simulink model "UrbanCHIL"  (Simulink 8.1)
settings: Solver=ode1  StartTime=0.0  StopTime=inf  FixedStep=Ts  MaxStep=1e-3  RelTol=1e-3
PostLoadFcn:
  | NREL_Mode=1; BANSHEE_init;
InitFcn:
  | NREL_Mode=1; BANSHEE_init;
values from neighbouring files (symbols this model uses):
  DER_REL = xlsread('DER_relay.xlsx')    [relay_settings_init.m]
  F0 = xlsread('F0_relay_banshee.xlsx')    [relay_settings_init.m]
  F2 = xlsread('F2_relay_banshee.xlsx')    [relay_settings_init.m]
  F3 = xlsread('F3_relay_banshee.xlsx')    [relay_settings_init.m]
  F4 = xlsread('F4_relay_nrel.xlsx')    [relay_settings_init.m]
  Ts = 100E-6    (= 0.0001)    [BANSHEE_init.m]    (also in Ghost_init.m)
undefined symbols (not defined in the file or in its folder): CBID, communications_lib, Feeder2_lib, Feeder3_lib, Feeder4_lib, generic_ethernet_cb, Left, relay_housing_lib, SM_UtilityService, SS_COMMUNICATION, SS_F2_RELAY_HOUSING, SS_F3_RELAY_HOUSING, SS_Feeder2, SS_Feeder3, SS_Feeder4, Stim, type, utility_service_lib, V
libraries: simulink x80, relay_modbus_lib x80, breaker_lib x46, rtio_generic_modbus x45, cables_lib x30, rtlab x22, Load_lib x21, powerlib x20, transformer_lib x19, ssn_lib x13, artemis x6, BESS_lib x4
(part 2 of 6)

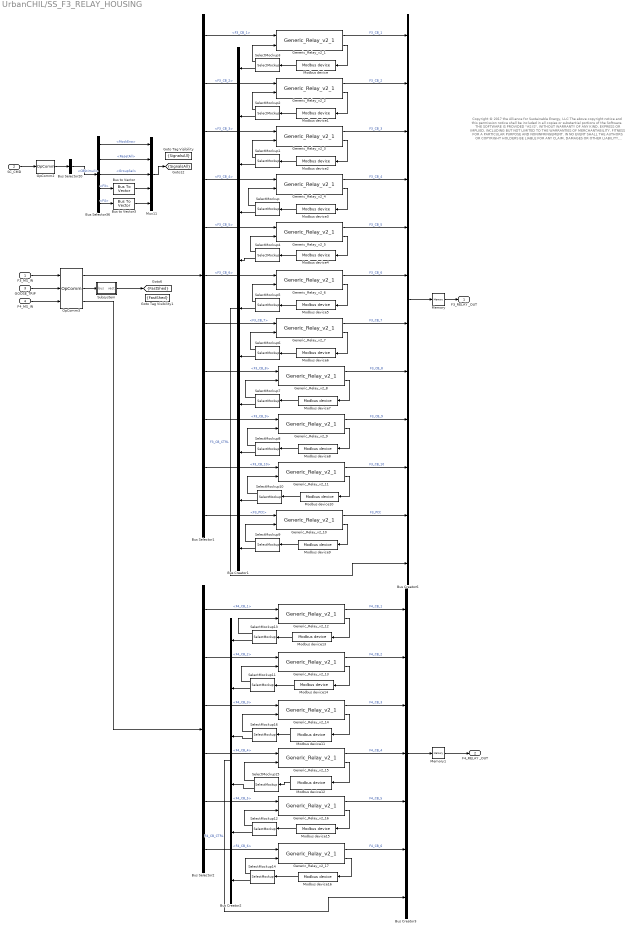
== system UrbanCHIL/SS_F3_RELAY_HOUSING ==
  note: Copyright © 2017 the Alliance for Sustainable Energy, LLC
      |
      | The above copyright notice and this permission notice shall be included in all copies or substantial portions of the Software.
      |
      | THE SOFTWARE IS PROVIDED "AS IS", WITHOUT WARRANTY OF ANY KIND, EXPRESS OR IMPLIED, INCLUDING
      | BUT NOT LIMITED TO THE WARRANTIES OF MERCHANTABILITY, FITNESS FOR A PARTICULAR PURPOSE AND
      | NONINFRINGEMENT. IN NO EVENT SHALL THE AUTHORS OR COPYRIGHT HOLDERS BE LIABLE FOR ANY CLAIM,
      |  DAMAGES OR OTHER LIABILITY, WHETHER IN AN ACTION OF CONTRACT, TORT OR OTHERWISE, ARISING FROM,
      | OUT OF OR IN CONNECTION WITH THE SOFTWARE OR THE USE OR OTHER DEALINGS IN THE SOFTWARE
  F3_MS_IN : Inport
  SC_CMD : Inport  Port=2
  GOOSE_TRIP : Inport  Port=3
  F4_MS_IN : Inport  Port=4
  Bus Creator1 : BusCreator  Inputs=11
  Bus Creator2 : BusCreator  Inputs=6
  Bus Creator3 : BusCreator  Inputs=7
  Bus Creator6 : BusCreator  Inputs=12
  Bus Selector1 : BusSelector  OutputSignals=CB_DATA.F3_CB_1,CB_DATA.F3_CB_2,CB_DATA.F3_CB_3,CB_DATA.F3_CB_4,CB_DATA.F3_CB_5,CB_DATA.F3_CB_6,CB_DATA.F3_CB_7,CB_DATA.F3_CB_8,CB_DATA.F3_CB_9,CB_DATA.F3_CB_10,CB_DATA.F3_PCC
  Bus Selector2 : BusSelector  OutputSignals=CB_DATA.F4_CB_1,CB_DATA.F4_CB_2,CB_DATA.F4_CB_3,CB_DATA.F4_CB_4,CB_DATA.F4_CB_5,CB_DATA.F4_CB_6
  Bus Selector20 : BusSelector  OutputSignals=CBStimuli
  Bus Selector36 : BusSelector  OutputSignals=MockEna,ResetAll,GroupSel,F3,F4
  Bus to Vector : BusToVector
  Bus to Vector3 : BusToVector
  Generic_Relay_v2_1 : relay_modbus_lib/Generic_Relay_v2_1  Ts=Ts  relay_settings=[F3(1,:)]
  Generic_Relay_v2_10 : relay_modbus_lib/Generic_Relay_v2_1  Ts=Ts  relay_settings=[F0(3,:)]
  Generic_Relay_v2_11 : relay_modbus_lib/Generic_Relay_v2_1  Ts=Ts  relay_settings=[F3(10,:)]
  Generic_Relay_v2_12 : relay_modbus_lib/Generic_Relay_v2_1  Ts=Ts  relay_settings=[F4(1,:)]
  Generic_Relay_v2_13 : relay_modbus_lib/Generic_Relay_v2_1  Ts=Ts  relay_settings=[F4(2,:)]
  Generic_Relay_v2_14 : relay_modbus_lib/Generic_Relay_v2_1  Ts=Ts  relay_settings=[F4(3,:)]
  Generic_Relay_v2_15 : relay_modbus_lib/Generic_Relay_v2_1  Ts=Ts  relay_settings=[F4(4,:)]
  Generic_Relay_v2_16 : relay_modbus_lib/Generic_Relay_v2_1  Ts=Ts  relay_settings=[F4(5,:)]
  Generic_Relay_v2_17 : relay_modbus_lib/Generic_Relay_v2_1  Ts=Ts  relay_settings=[F4(6,:)]
  Generic_Relay_v2_2 : relay_modbus_lib/Generic_Relay_v2_1  Ts=Ts  relay_settings=[F3(2,:)]
  Generic_Relay_v2_3 : relay_modbus_lib/Generic_Relay_v2_1  Ts=Ts  relay_settings=[F3(3,:)]
  Generic_Relay_v2_4 : relay_modbus_lib/Generic_Relay_v2_1  Ts=Ts  relay_settings=[F3(4,:)]
  Generic_Relay_v2_5 : relay_modbus_lib/Generic_Relay_v2_1  Ts=Ts  relay_settings=[F3(5,:)]
  Generic_Relay_v2_6 : relay_modbus_lib/Generic_Relay_v2_1  Ts=Ts  relay_settings=[F3(6,:)]
  Generic_Relay_v2_7 : relay_modbus_lib/Generic_Relay_v2_1  Ts=Ts  relay_settings=[F3(7,:)]
  Generic_Relay_v2_8 : relay_modbus_lib/Generic_Relay_v2_1  Ts=Ts  relay_settings=[F3(8,:)]
  Generic_Relay_v2_9 : relay_modbus_lib/Generic_Relay_v2_1  Ts=Ts  relay_settings=[F3(9,:)]
  Goto Tag Visibility : GotoTagVisibility  GotoTag=SignalsAll
  Goto Tag Visibility1 : GotoTagVisibility  GotoTag=FastShed
  Memory : Memory
  Memory1 : Memory
  Modbus device : rtio_generic_modbus/Modbus device  conf_name=F3_relay_cfg1.opal  conf_name_mask=F3_relay_cfg1.xls  sample_time=Ts
  Modbus device1 : rtio_generic_modbus/Modbus device  conf_name=F3_relay_cfg2.opal  conf_name_mask=F3_relay_cfg2.xls  sample_time=Ts
  Modbus device10 : rtio_generic_modbus/Modbus device  conf_name=F3_relay_cfg10.opal  conf_name_mask=F3_relay_cfg10.xls  sample_time=Ts
  Modbus device11 : rtio_generic_modbus/Modbus device  conf_name=F4_relay_cfg3.opal  conf_name_mask=F4_relay_cfg3.xls  sample_time=Ts
  Modbus device12 : rtio_generic_modbus/Modbus device  conf_name=F4_relay_cfg4.opal  conf_name_mask=F4_relay_cfg4.xls  sample_time=Ts
  Modbus device13 : rtio_generic_modbus/Modbus device  conf_name=F4_relay_cfg1.opal  conf_name_mask=F4_relay_cfg1.xls  sample_time=Ts
  Modbus device14 : rtio_generic_modbus/Modbus device  conf_name=F4_relay_cfg2.opal  conf_name_mask=F4_relay_cfg2.xls  sample_time=Ts
  Modbus device15 : rtio_generic_modbus/Modbus device  conf_name=F4_relay_cfg5.opal  conf_name_mask=F4_relay_cfg5.xls  sample_time=Ts
  Modbus device16 : rtio_generic_modbus/Modbus device  conf_name=F4_relay_cfg6.opal  conf_name_mask=F4_relay_cfg6.xls  sample_time=Ts
  Modbus device2 : rtio_generic_modbus/Modbus device  conf_name=F3_relay_cfg3.opal  conf_name_mask=F3_relay_cfg3.xls  sample_time=Ts
  Modbus device3 : rtio_generic_modbus/Modbus device  conf_name=F3_relay_cfg4.opal  conf_name_mask=F3_relay_cfg4.xls  sample_time=Ts
  Modbus device4 : rtio_generic_modbus/Modbus device  conf_name=F3_relay_cfg5.opal  conf_name_mask=F3_relay_cfg5.xls  sample_time=Ts
  Modbus device5 : rtio_generic_modbus/Modbus device  conf_name=F3_relay_cfg6.opal  conf_name_mask=F3_relay_cfg6.xls  sample_time=Ts
  Modbus device6 : rtio_generic_modbus/Modbus device  conf_name=F3_relay_cfg7.opal  conf_name_mask=F3_relay_cfg7.xls  sample_time=Ts
  Modbus device7 : rtio_generic_modbus/Modbus device  conf_name=F3_relay_cfg8.opal  conf_name_mask=F3_relay_cfg8.xls  sample_time=Ts
  Modbus device8 : rtio_generic_modbus/Modbus device  conf_name=F3_relay_cfg9.opal  conf_name_mask=F3_relay_cfg9.xls  sample_time=Ts
  Modbus device9 : rtio_generic_modbus/Modbus device  conf_name=F3_relay_cfg_pcc.opal  conf_name_mask=F3_relay_cfg_pcc.xls  sample_time=Ts
  Mux11 : Mux  Inputs=5
  OpComm2 : rtlab/OpComm  nbport=1  groupe_acq=1  subsys_rate=0  st=0  Synchronization=on  Interpolation=on  Threshold=1.0  Missed_Data=off  Sim_Time=off  Samples=off  dynSigOut=off  from_console=0  warning_done=off  writeOpCommFile=off  Offset=off
  OpComm3 : rtlab/OpComm  nbport=3  groupe_acq=1  subsys_rate=0  st=0  Synchronization=on  Interpolation=on  Threshold=1.0  Missed_Data=off  Sim_Time=off  Samples=off  dynSigOut=off  from_console=0  warning_done=off  writeOpCommFile=off  Offset=off
  SelectMockup : relay_modbus_lib/SelectMockup  sigID=4  sigN=17
  SelectMockup1 : relay_modbus_lib/SelectMockup  sigID=3  sigN=17
  SelectMockup10 : relay_modbus_lib/SelectMockup  sigID=10  sigN=17
  SelectMockup11 : relay_modbus_lib/SelectMockup  sigID=13  sigN=17
  SelectMockup12 : relay_modbus_lib/SelectMockup  sigID=16  sigN=17
  SelectMockup13 : relay_modbus_lib/SelectMockup  sigID=12  sigN=17
  SelectMockup14 : relay_modbus_lib/SelectMockup  sigID=17  sigN=17
  SelectMockup15 : relay_modbus_lib/SelectMockup  sigID=15  sigN=17
  SelectMockup16 : relay_modbus_lib/SelectMockup  sigID=14  sigN=17
  SelectMockup2 : relay_modbus_lib/SelectMockup  sigID=2  sigN=17
  SelectMockup3 : relay_modbus_lib/SelectMockup  sigID=1  sigN=17
  SelectMockup4 : relay_modbus_lib/SelectMockup  sigID=5  sigN=17
  SelectMockup5 : relay_modbus_lib/SelectMockup  sigID=6  sigN=17
  SelectMockup6 : relay_modbus_lib/SelectMockup  sigID=7  sigN=17
  SelectMockup7 : relay_modbus_lib/SelectMockup  sigID=8  sigN=17
  SelectMockup8 : relay_modbus_lib/SelectMockup  sigID=9  sigN=17
  SelectMockup9 : relay_modbus_lib/SelectMockup  sigID=11  sigN=17
  Subsystem : Subsystem
  F3_RELAY _OUT : Outport
  F4_RELAY _OUT : Outport  Port=2
  tag scope: FastShed=scoped, SignalsAll=scoped
  wires:
  OpComm3/1 -> Bus Selector1/1
  Generic_Relay_v2_1/2 -> Modbus device/1
  SelectMockup3/1 -> Generic_Relay_v2_1/2
  Generic_Relay_v2_2/2 -> Modbus device1/1
  SelectMockup2/1 -> Generic_Relay_v2_2/2
  SelectMockup1/1 -> Generic_Relay_v2_3/2
  Generic_Relay_v2_3/2 -> Modbus device2/1
  Generic_Relay_v2_4/2 -> Modbus device3/1
  SelectMockup/1 -> Generic_Relay_v2_4/2
  Generic_Relay_v2_5/2 -> Modbus device4/1
  SelectMockup4/1 -> Generic_Relay_v2_5/2
  SelectMockup5/1 -> Generic_Relay_v2_6/2
  Generic_Relay_v2_6/2 -> Modbus device5/1
  Generic_Relay_v2_7/2 -> Modbus device6/1
  SelectMockup6/1 -> Generic_Relay_v2_7/2
  F3_MS_IN/1 -> OpComm3/1
  Bus Selector1/1 -> Generic_Relay_v2_1/1  "<F3_CB_1>"
  Bus Selector1/2 -> Generic_Relay_v2_2/1  "<F3_CB_2>"
  Bus Selector1/3 -> Generic_Relay_v2_3/1  "<F3_CB_3>"
  Bus Selector1/4 -> Generic_Relay_v2_4/1  "<F3_CB_4>"
  Bus Selector1/5 -> Generic_Relay_v2_5/1  "<F3_CB_5>"
  Bus Selector1/6 -> Generic_Relay_v2_6/1  "<F3_CB_6>"
  Bus Selector1/7 -> Generic_Relay_v2_7/1  "<F3_CB_7>"
  Generic_Relay_v2_1/1 -> Bus Creator6/1  "F3_CB_1"
  Generic_Relay_v2_2/1 -> Bus Creator6/2  "F3_CB_2"
  Generic_Relay_v2_3/1 -> Bus Creator6/3  "F3_CB_3"
  Generic_Relay_v2_4/1 -> Bus Creator6/4  "F3_CB_4"
  Generic_Relay_v2_5/1 -> Bus Creator6/5  "F3_CB_5"
  Generic_Relay_v2_6/1 -> Bus Creator6/6  "F3_CB_6"
  Generic_Relay_v2_7/1 -> Bus Creator6/7  "F3_CB_7"
  Bus Creator6/1 -> Memory/1
  SelectMockup7/1 -> Generic_Relay_v2_8/2
  Generic_Relay_v2_8/2 -> Modbus device7/1
  Generic_Relay_v2_9/2 -> Modbus device8/1
  SelectMockup8/1 -> Generic_Relay_v2_9/2
  Generic_Relay_v2_8/1 -> Bus Creator6/8  "F3_CB_8"
  Generic_Relay_v2_9/1 -> Bus Creator6/9  "F3_CB_9"
  Bus Selector1/9 -> Generic_Relay_v2_9/1  "<F3_CB_9>"
  Bus Selector1/8 -> Generic_Relay_v2_8/1  "<F3_CB_8>"
  Memory/1 -> F3_RELAY _OUT/1
  Generic_Relay_v2_10/1 -> Bus Creator6/11  "F3_PCC"
  Generic_Relay_v2_10/2 -> Modbus device9/1
  SelectMockup9/1 -> Generic_Relay_v2_10/2
  Bus Selector1/10 -> Generic_Relay_v2_11/1  "<F3_CB_10>"
  SC_CMD/1 -> OpComm2/1
  OpComm2/1 -> Bus Selector20/1
  Bus Selector20/1 -> Bus Selector36/1  "<CBStimuli>"
  Bus Selector36/4 -> Bus to Vector/1  "<F3>"
  Bus Selector36/1 -> Mux11/1  "<MockEna>"
  Bus to Vector/1 -> Mux11/4
  Bus Selector36/3 -> Mux11/3  "<GroupSel>"
  Bus Selector36/2 -> Mux11/2  "<ResetAll>"
  Mux11/1 -> [SignalsAll]
  Modbus device9/1 -> SelectMockup9/1
  Modbus device8/1 -> SelectMockup8/1
  Modbus device7/1 -> SelectMockup7/1
  Modbus device6/1 -> SelectMockup6/1
  Modbus device5/1 -> SelectMockup5/1
  Modbus device4/1 -> SelectMockup4/1
  Modbus device3/1 -> SelectMockup/1
  Modbus device1/1 -> SelectMockup2/1
  Modbus device/1 -> SelectMockup3/1
  Modbus device2/1 -> SelectMockup1/1
  Generic_Relay_v2_11/1 -> Bus Creator6/10  "F3_CB_10"
  Generic_Relay_v2_11/2 -> Modbus device10/1
  SelectMockup10/1 -> Generic_Relay_v2_11/2
  Modbus device10/1 -> SelectMockup10/1
  Bus Selector1/11 -> Generic_Relay_v2_10/1  "<F3_PCC>"
  GOOSE_TRIP/1 -> OpComm3/2
  OpComm3/2 -> Subsystem/1(bus)
  Subsystem/1(vect) -> [FastShed]
  SelectMockup3/2 -> Bus Creator1/1
  SelectMockup2/2 -> Bus Creator1/2
  SelectMockup1/2 -> Bus Creator1/3
  SelectMockup/2 -> Bus Creator1/4
  SelectMockup4/2 -> Bus Creator1/5
  SelectMockup5/2 -> Bus Creator1/6
  SelectMockup6/2 -> Bus Creator1/7
  SelectMockup7/2 -> Bus Creator1/8
  SelectMockup8/2 -> Bus Creator1/9
  SelectMockup10/2 -> Bus Creator1/10
  SelectMockup9/2 -> Bus Creator1/11
  Bus Creator1/1 -> Bus Creator6/12  "F3_CB_CTRL"
  Modbus device11/1 -> SelectMockup16/1
  SelectMockup16/1 -> Generic_Relay_v2_14/2
  SelectMockup15/1 -> Generic_Relay_v2_15/2
  Modbus device12/1 -> SelectMockup15/1
  SelectMockup14/1 -> Generic_Relay_v2_17/2
  Modbus device16/1 -> SelectMockup14/1
  Generic_Relay_v2_17/2 -> Modbus device16/1
  SelectMockup12/1 -> Generic_Relay_v2_16/2
  Modbus device15/1 -> SelectMockup12/1
  Generic_Relay_v2_16/2 -> Modbus device15/1
  SelectMockup11/1 -> Generic_Relay_v2_13/2
  Modbus device14/1 -> SelectMockup11/1
  Generic_Relay_v2_13/2 -> Modbus device14/1
  SelectMockup13/1 -> Generic_Relay_v2_12/2
  Modbus device13/1 -> SelectMockup13/1
  Generic_Relay_v2_15/2 -> Modbus device12/1
  Generic_Relay_v2_14/2 -> Modbus device11/1
  Memory1/1 -> F4_RELAY _OUT/1
  Bus Creator3/1 -> Memory1/1
  Generic_Relay_v2_17/1 -> Bus Creator3/6  "F4_CB_6"
  Generic_Relay_v2_16/1 -> Bus Creator3/5  "F4_CB_5"
  Generic_Relay_v2_15/1 -> Bus Creator3/4  "F4_CB_4"
  Generic_Relay_v2_14/1 -> Bus Creator3/3  "F4_CB_3"
  Generic_Relay_v2_13/1 -> Bus Creator3/2  "F4_CB_2"
  Generic_Relay_v2_12/1 -> Bus Creator3/1  "F4_CB_1"
  Bus Selector2/6 -> Generic_Relay_v2_17/1  "<F4_CB_6>"
  Bus Selector2/5 -> Generic_Relay_v2_16/1  "<F4_CB_5>"
  Bus Selector2/4 -> Generic_Relay_v2_15/1  "<F4_CB_4>"
  Bus Selector2/3 -> Generic_Relay_v2_14/1  "<F4_CB_3>"
  Bus Selector2/2 -> Generic_Relay_v2_13/1  "<F4_CB_2>"
  Bus Selector2/1 -> Generic_Relay_v2_12/1  "<F4_CB_1>"
  F4_MS_IN/1 -> OpComm3/3
  Generic_Relay_v2_12/2 -> Modbus device13/1
  OpComm3/3 -> Bus Selector2/1
  SelectMockup13/2 -> Bus Creator2/1
  SelectMockup11/2 -> Bus Creator2/2
  SelectMockup16/2 -> Bus Creator2/3
  SelectMockup15/2 -> Bus Creator2/4
  SelectMockup12/2 -> Bus Creator2/5
  SelectMockup14/2 -> Bus Creator2/6
  Bus Creator2/1 -> Bus Creator3/7  "F4_CB_CTRL"
  Bus Selector36/5 -> Bus to Vector3/1  "<F4>"
  Bus to Vector3/1 -> Mux11/5

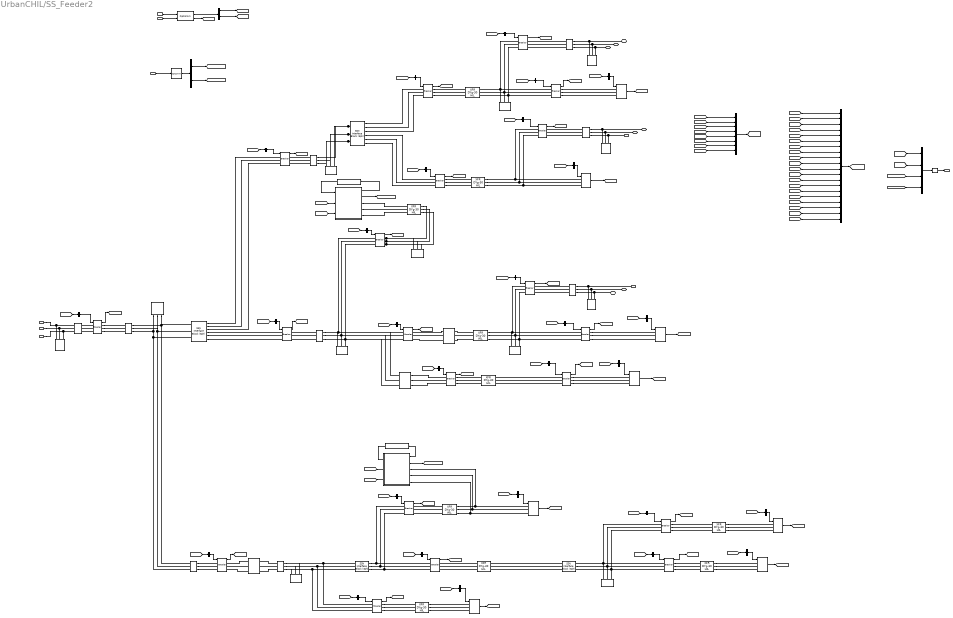
== system UrbanCHIL/SS_Feeder2 ==
  note: connect to F3
  note: connect to F3
  note: connect to F3
  note: PV SYSTEM
  note: % Copyright (c) 2016 Massachusetts Institute of Technology
      | % Permission is hereby granted, free of charge, to any person obtaining a copy of this
      | % software and associated documentation files (the "Software"), to deal in the Software
      | % without restriction, including without limitation the rights to use, copy, modify,
      | % merge, publish, distribute, sublicense, and/or sell copies of the Software, and to
      | % permit persons to whom the Software is furnished to do so, subject to the following
      | % conditions:
      | %
      | %
      | % The above copyright notice and this permission notice shall be included in
      | % all copies or substantial portions of the Software.
      | %
      | % THE SOFTWARE IS PROVIDED "AS IS", WITHOUT WARRANTY OF ANY KIND, EXPRESS OR IMPLIED,
      | % INCLUDING BUT NOT LIMITED TO THE WARRANTIES OF MERCHANTABILITY, FITNESS FOR A
      | % PARTICULAR PURPOSE AND NONINFRINGEMENT. IN NO EVENT SHALL THE AUTHORS OR COPYRIGHT
      | % HOLDERS BE LIABLE FOR ANY CLAIM, DAMAGES OR OTHER LIABILITY, WHETHER IN AN ACTION
      | % OF CONTRACT, TORT OR OTHERWISE, ARISING FROM, OUT OF OR IN CONNECTION WITH THE
      | % SOFTWARE OR THE USE OR OTHER DEALINGS IN THE SOFTWARE.
      | %
      | %
      | %%
  note: BESS SYSTEM
  RELAY_IN : Inport
  LOAD_IN : Inport  Port=2
  SC_CMD : Inport  Port=3
  1000 kVA1 : transformer_lib/XFR DYg-30 HIL  Rating=1000  Vp=13800  Vs=480  Z=5.56  XR=4.49
  1000 kVA2 : transformer_lib/XFR DYg-30 HIL  Rating=1000  Vp=4160  Vs=480  Z=5.56  XR=5.49
  1500 kVA : transformer_lib/XFR DYg-30 HIL  Rating=1500  Vp=4160  Vs=480  Z=5.56  XR=5.51
  2000 kVA2 : transformer_lib/XFR DYg-30 HIL  Rating=2000  Vp=13800  Vs=480  Z=5.75  XR=5.7
  2000 kVA3 : transformer_lib/XFR DYg-30 HIL  Rating=2000  Vp=13800  Vs=480  Z=5.75  XR=5.7
  2500 kVA : transformer_lib/XFR DYg-30 HIL  Rating=2500  Vp=13800  Vs=480  Z=5.56  XR=5.52
  2500 kVA1 : transformer_lib/XFR DYg-30 HIL  Rating=2500  Vp=13800  Vs=480  Z=5.56  XR=5.52
  3750 kVA : transformer_lib/XFR DYg-30 HIL  Rating=3750  Vp=13800  Vs=4160  Z=4.75  XR=11.4
  4/0AWG-Mutual : cables_lib/4//0AWG-Mutual  length=10  par_sets=1  ratio=3
  448 kvar inductor at 13.8kV  to cancel kvar produced by the stublines1 : powerlib/Elements/Three-Phase Parallel RLC Load  LConnTagsString=A|B|C  Configuration=Y (grounded)  NominalVoltage=13800  NominalFrequency=60  ActivePower=10e3  InductivePower=448e3  CapacitivePower=0  Measurements=None  LoadType=constant Z
  500 kVA : transformer_lib/XFR DYg-30 HIL  Rating=500  Vp=13800  Vs=208  Z=5  XR=4.9
  5000 kVA : transformer_lib/XFR DYg-30 HIL  Rating=5000  Vp=13800  Vs=480  Z=3  XR=5.44
  500kcmil-Mutual5 : cables_lib/500kcmil-Mutual  length=1000  par_sets=1  ratio=3
  500kcmil-Mutual8 : cables_lib/500kcmil-Mutual  length=100  par_sets=1  ratio=3
  6 kvar inductor at 480V  to cancel kvar produced by the stublines1 : powerlib/Elements/Three-Phase Parallel RLC Load  LConnTagsString=A|B|C  Configuration=Y (grounded)  NominalVoltage=480  NominalFrequency=60  ActivePower=1e3  InductivePower=6e3  CapacitivePower=0  Measurements=None  LoadType=constant Z
  6 kvar inductor at 480V  to cancel kvar produced by the stublines2 : powerlib/Elements/Three-Phase Parallel RLC Load  LConnTagsString=A|B|C  Configuration=Y (grounded)  NominalVoltage=480  NominalFrequency=60  ActivePower=1e3  InductivePower=6e3  CapacitivePower=0  Measurements=None  LoadType=constant Z
  6 kvar inductor at 480V  to cancel kvar produced by the stublines3 : powerlib/Elements/Three-Phase Parallel RLC Load  LConnTagsString=A|B|C  Configuration=Y (grounded)  NominalVoltage=480  NominalFrequency=60  ActivePower=1  InductivePower=6e3  CapacitivePower=0  Measurements=None  LoadType=constant Z
  Bus Creator2 : BusCreator
  Bus Creator3 : BusCreator  Inputs=8
  Bus Creator5 : BusCreator  Inputs=20
  Bus Selector1 : BusSelector  OutputSignals=F2_CB_4
  Bus Selector10 : BusSelector  OutputSignals=I4
  Bus Selector11 : BusSelector  OutputSignals=F2_CB_11
  Bus Selector12 : BusSelector  OutputSignals=F2_CB_15
  Bus Selector13 : BusSelector  OutputSignals=F2_CB_3
  Bus Selector14 : BusSelector  OutputSignals=F2_CB_14
  Bus Selector15 : BusSelector  OutputSignals=F2_CB_17
  Bus Selector16 : BusSelector  OutputSignals=F2_CB_16
  Bus Selector17 : BusSelector  OutputSignals=F2_CB_13
  Bus Selector18 : BusSelector  OutputSignals=F2_CB_10
  Bus Selector19 : BusSelector  OutputSignals=F2_CB_9
  Bus Selector2 : BusSelector  OutputSignals=F2_CB_2
  Bus Selector20 : BusSelector  OutputSignals=F2_CB_12
  Bus Selector21 : BusSelector  OutputSignals=F2_CB_5
  Bus Selector22 : BusSelector  OutputSignals=F2_CB_7
  Bus Selector23 : BusSelector  OutputSignals=F2_CB_8
  Bus Selector24 : BusSelector  OutputSignals=F2_CB_6
  Bus Selector25 : BusSelector  OutputSignals=F2_CB_1
  Bus Selector26 : BusSelector  OutputSignals=F2_CB_18
  Bus Selector27 : BusSelector  OutputSignals=F2_CB_19
  Bus Selector28 : BusSelector  OutputSignals=ESS1_ctrl,PV1_ctrl
  Bus Selector3 : BusSelector  OutputSignals=P5
  Bus Selector30 : BusSelector  OutputSignals=LoadProfile,TestSeq
  Bus Selector36 : BusSelector  OutputSignals=F2_PCC
  Bus Selector4 : BusSelector  OutputSignals=C4
  Bus Selector5 : BusSelector  OutputSignals=I5
  Bus Selector6 : BusSelector  OutputSignals=P2
  Bus Selector7 : BusSelector  OutputSignals=C3
  Bus Selector8 : BusSelector  OutputSignals=P3
  Bus Selector9 : BusSelector  OutputSignals=I3
  C201 : cables_lib/4//0AWG-Mutual  length=5500  par_sets=1  ratio=3
  C202 : cables_lib/500kcmil-Mutual  length=2000  par_sets=1  ratio=3
  C203 : cables_lib/500kcmil-Mutual  length=3000  par_sets=1  ratio=3
  C204 : cables_lib/500kcmil-Mutual  length=10  par_sets=1  ratio=3
  C205 : cables_lib/500kcmil-Mutual  length=10  par_sets=1  ratio=3
  C206 : cables_lib/500kcmil-Mutual  length=10  par_sets=1  ratio=3
  Critical_3 : Load_lib/Dynamic_Load  V=480  kVA=1000  PF=0.9  Ts=Ts
  Critical_4 : Load_lib/Dynamic_Load  V=480  kVA=1000  PF=0.9  Ts=Ts
  ESS1 : Subsystem
  ESS1_Modbus : rtio_generic_modbus/Modbus device  conf_name=ESS1_modbus.opal  conf_name_mask=ESS1_modbus.xls  sample_time=Ts
  F2_CB_{1..19} (19 alike) : breaker_lib/Breaker  Ts=Ts  mech_delay=cb_mech_delay
  F2_PCC : breaker_lib/Breaker  Ts=Ts  mech_delay=cb_mech_delay
  Interruptible_3 : Load_lib/Dynamic_Load  V=208  kVA=300  PF=0.9  Ts=Ts
  Interruptible_4 : Load_lib/Dynamic_Load  V=480  kVA=600  PF=0.9  Ts=Ts
  Interruptible_5 : Load_lib/Dynamic_Load  V=480  kVA=400  PF=0.9  Ts=Ts
  Losses{1,3..4,6,8} (5 alike) : powerlib/Elements/Three-Phase Parallel RLC Load  LConnTagsString=A|B|C  Configuration=Y (grounded)  NominalVoltage=13800  NominalFrequency=60  ActivePower=1e3  InductivePower=0  CapacitivePower=0  Measurements=None  LoadType=constant Z
  Losses2 : powerlib/Elements/Three-Phase Parallel RLC Load  LConnTagsString=A|B|C  Configuration=Y (grounded)  NominalVoltage=480  NominalFrequency=60  ActivePower=1e3  InductivePower=0  CapacitivePower=0  Measurements=None  LoadType=constant Z
  Losses5 : powerlib/Elements/Three-Phase Parallel RLC Load  LConnTagsString=A|B|C  Configuration=Y (grounded)  NominalVoltage=480  NominalFrequency=60  ActivePower=1e3  InductivePower=0  CapacitivePower=0  Measurements=None  LoadType=constant Z
  Losses7 : powerlib/Elements/Three-Phase Parallel RLC Load  LConnTagsString=A|B|C  Configuration=Y (grounded)  NominalVoltage=4160  NominalFrequency=60  ActivePower=1e3  InductivePower=0  CapacitivePower=0  Measurements=None  LoadType=constant Z
  Memory : Memory
  OpComm1 : rtlab/OpComm  nbport=2  groupe_acq=1  subsys_rate=0  st=0  Synchronization=on  Interpolation=on  Threshold=1.0  Missed_Data=off  Sim_Time=off  Samples=off  dynSigOut=off  from_console=0  warning_done=off  writeOpCommFile=off  Offset=off
  OpComm2 : rtlab/OpComm  nbport=1  groupe_acq=1  subsys_rate=0  st=0  Synchronization=on  Interpolation=on  Threshold=1.0  Missed_Data=off  Sim_Time=off  Samples=off  dynSigOut=off  from_console=1  warning_done=off  writeOpCommFile=off  Offset=off
  PV1_Modbus : rtio_generic_modbus/Modbus device  conf_name=PV1_modbus.opal  conf_name_mask=PV1_modbus.xls  sample_time=Ts
  PV2 : Subsystem
  Priority_2 : Load_lib/Dynamic_Load  V=480  kVA=1000  PF=0.9  Ts=Ts
  Priority_3 : Load_lib/Dynamic_Load  V=480  kVA=1000  PF=0.9  Ts=Ts
  Priority_5 : Load_lib/Dynamic_Load  V=480  kVA=700  PF=0.9  Ts=Ts
  SSN Interface Block (3ph){1,3,5,9..10} (5 alike) : ssn_lib/SSN Interface Block (3ph)  nb_phase=3  nb_port=2  p1_type=V-type(Left)  p2_type=V-type (Right)  p3_type=V-type(Left)  p4_type=V-type(Left)  p5_type=V-type(Left)  p6_type=V-type(Left)  p7_type=V-type(Left)  p8_type=V-type(Left)  p9_type=V-type(Left)  p10_type=V-type(Left)  p11_type=V-type(Left)  p12_type=V-type(Left)  p13_type=V-type(Left)  p14_type=V-type(Left)  p15_type=V-type(Left)  p16_type=V-type(Left)  I_port_shunt_resistance=1e9
  SSN Interface Block (3ph)2 : ssn_lib/SSN Interface Block (3ph)  nb_phase=3  nb_port=3  p1_type=V-type(Left)  p2_type=V-type (Right)  p3_type=V-type (Right)  p4_type=V-type(Left)  p5_type=V-type(Left)  p6_type=V-type(Left)  p7_type=V-type(Left)  p8_type=V-type(Left)  p9_type=V-type(Left)  p10_type=V-type(Left)  p11_type=V-type(Left)  p12_type=V-type(Left)  p13_type=V-type(Left)  p14_type=V-type(Left)  p15_type=V-type(Left)  p16_type=V-type(Left)  I_port_shunt_resistance=1e9
  SSN Interface Block (3ph)4 : ssn_lib/SSN Interface Block (3ph)  nb_phase=3  nb_port=3  p1_type=V-type(Left)  p2_type=V-type (Right)  p3_type=V-type (Right)  p4_type=V-type(Left)  p5_type=V-type(Left)  p6_type=V-type(Left)  p7_type=V-type(Left)  p8_type=V-type(Left)  p9_type=V-type(Left)  p10_type=V-type(Left)  p11_type=V-type(Left)  p12_type=V-type(Left)  p13_type=V-type(Left)  p14_type=V-type(Left)  p15_type=V-type(Left)  p16_type=V-type(Left)  I_port_shunt_resistance=1e9
  A_CB_13 : PMIOPort  Port=1  Side=Right
  B_CB_13 : PMIOPort  Port=2  Side=Right
  C_CB_13 : PMIOPort  Port=3  Side=Right
  A_CB_17 : PMIOPort  Port=4  Side=Right
  B_CB_17 : PMIOPort  Port=5  Side=Right
  C_CB_17 : PMIOPort  Port=6  Side=Right
  A_CB_16 : PMIOPort  Port=7  Side=Right
  B_CB_16 : PMIOPort  Port=8  Side=Right
  C_CB_16 : PMIOPort  Port=9  Side=Right
  PCC_A : PMIOPort  Port=10  Side=Left
  PCC_B : PMIOPort  Port=11  Side=Left
  PCC_C : PMIOPort  Port=12  Side=Left
  DATA_OUT : Outport
  wires:
  LOAD_IN/1 -> OpComm1/1
  [LOAD_IN] -> Bus Selector3/1
  [LOAD_IN] -> Bus Selector4/1
  [LOAD_IN] -> Bus Selector5/1
  [LOAD_IN] -> Bus Selector6/1
  [LOAD_IN] -> Bus Selector7/1
  [LOAD_IN] -> Bus Selector8/1
  [LOAD_IN] -> Bus Selector9/1
  [LOAD_IN] -> Bus Selector10/1
  Bus Selector3/1 -> Priority_5/1  "<P5>"
  Bus Selector4/1 -> Critical_4/1  "<C4>"
  Bus Selector5/1 -> Interruptible_5/1  "<I5>"
  Bus Selector6/1 -> Priority_2/1  "<P2>"
  Bus Selector7/1 -> Critical_3/1  "<C3>"
  Bus Selector8/1 -> Priority_3/1  "<P3>"
  Bus Selector10/1 -> Interruptible_4/1  "<I4>"
  Bus Selector9/1 -> Interruptible_3/1  "<I3>"
  Critical_4/1 -> [LOAD_C4]
  Priority_5/1 -> [LOAD_P5]
  Interruptible_5/1 -> [LOAD_I5]
  Priority_2/1 -> [LOAD_P2]
  Critical_3/1 -> [LOAD_C3]
  Interruptible_3/1 -> [LOAD_I3]
  Priority_3/1 -> [LOAD_P3]
  Interruptible_4/1 -> [LOAD_I4]
  [LOAD_C3] -> Bus Creator3/1  "F2_C3"
  Bus Creator3/1 -> [LOAD_DATA]  "LOAD"
  [LOAD_I4] -> Bus Creator3/4  "F2_I4"
  [LOAD_P2] -> Bus Creator3/6  "F2_P2"
  [LOAD_I5] -> Bus Creator3/5  "F2_I5"
  [LOAD_C4] -> Bus Creator3/2  "F2_C4"
  [LOAD_I3] -> Bus Creator3/3  "F2_I3"
  [LOAD_P3] -> Bus Creator3/7  "F2_P3"
  [LOAD_P5] -> Bus Creator3/8  "F2_P5"
  F2_CB_2/1 -> [F2_CB_2]
  F2_CB_1/1 -> [F2_CB_1]
  F2_CB_6/1 -> [F2_CB_6]
  F2_CB_7/1 -> [F2_CB_7]
  F2_CB_5/1 -> [F2_CB_5]
  F2_CB_8/1 -> [F2_CB_8]
  F2_CB_9/1 -> [F2_CB_9]
  F2_CB_3/1 -> [F2_CB_3]
  F2_CB_11/1 -> [F2_CB_11]
  F2_CB_15/1 -> [F2_CB_15]
  F2_CB_17/1 -> [F2_CB_17]
  F2_CB_14/1 -> [F2_CB_14]
  F2_CB_10/1 -> [F2_CB_10]
  F2_CB_13/1 -> [F2_CB_13]
  [F2_CB_1] -> Bus Creator5/1  "F2_CB_1"
  [F2_CB_2] -> Bus Creator5/2  "F2_CB_2"
  [F2_CB_3] -> Bus Creator5/3  "F2_CB_3"
  [F2_CB_6] -> Bus Creator5/6  "F2_CB_6"
  [F2_CB_4] -> Bus Creator5/4  "F2_CB_4"
  [F2_CB_9] -> Bus Creator5/9  "F2_CB_9"
  [F2_CB_7] -> Bus Creator5/7  "F2_CB_7"
  [F2_CB_11] -> Bus Creator5/11  "F2_CB_11"
  [F2_CB_14] -> Bus Creator5/14  "F2_CB_14"
  [F2_CB_5] -> Bus Creator5/5  "F2_CB_5"
  [F2_CB_8] -> Bus Creator5/8  "F2_CB_8"
  [F2_CB_12] -> Bus Creator5/12  "F2_CB_12"
  [F2_CB_10] -> Bus Creator5/10  "F2_CB_10"
  [F2_CB_13] -> Bus Creator5/13  "F2_CB_13"
  [F2_CB_15] -> Bus Creator5/15  "F2_CB_15"
  [F2_CB_16] -> Bus Creator5/16  "F2_CB_16"
  RELAY_IN/1 -> OpComm1/2
  OpComm1/2 -> [RELAY_IN]
  Bus Selector13/1 -> F2_CB_3/1  "<F2_CB_3>"
  [RELAY_IN] -> Bus Selector13/1
  [RELAY_IN] -> Bus Selector2/1
  [RELAY_IN] -> Bus Selector11/1
  [RELAY_IN] -> Bus Selector12/1
  [RELAY_IN] -> Bus Selector14/1
  [RELAY_IN] -> Bus Selector15/1
  [RELAY_IN] -> Bus Selector16/1
  [RELAY_IN] -> Bus Selector17/1
  [RELAY_IN] -> Bus Selector18/1
  [RELAY_IN] -> Bus Selector19/1
  [RELAY_IN] -> Bus Selector20/1
  [RELAY_IN] -> Bus Selector21/1
  [RELAY_IN] -> Bus Selector22/1
  [RELAY_IN] -> Bus Selector23/1
  [RELAY_IN] -> Bus Selector24/1
  [RELAY_IN] -> Bus Selector25/1
  Bus Selector2/1 -> F2_CB_2/1  "<F2_CB_2>"
  Bus Selector11/1 -> F2_CB_11/1  "<F2_CB_11>"
  Bus Selector18/1 -> F2_CB_10/1  "<F2_CB_10>"
  Bus Selector19/1 -> F2_CB_9/1  "<F2_CB_9>"
  Bus Selector17/1 -> F2_CB_13/1  "<F2_CB_13>"
  Bus Selector20/1 -> F2_CB_12/1  "<F2_CB_12>"
  Bus Selector14/1 -> F2_CB_14/1  "<F2_CB_14>"
  Bus Selector16/1 -> F2_CB_16/1  "<F2_CB_16>"
  Bus Selector12/1 -> F2_CB_15/1  "<F2_CB_15>"
  Bus Selector25/1 -> F2_CB_1/1  "<F2_CB_1>"
  Bus Selector21/1 -> F2_CB_5/1  "<F2_CB_5>"
  Bus Selector22/1 -> F2_CB_7/1  "<F2_CB_7>"
  Bus Selector24/1 -> F2_CB_6/1  "<F2_CB_6>"
  Bus Selector23/1 -> F2_CB_8/1  "<F2_CB_8>"
  [F2_CB_17] -> Bus Creator5/17  "F2_CB_17"
  Bus Selector15/1 -> F2_CB_17/1  "<F2_CB_17>"
  F2_CB_12/1 -> [F2_CB_12]
  F2_CB_16/1 -> [F2_CB_16]
  F2_PCC/1 -> [F2_PCC]
  [F2_PCC] -> Bus Creator5/20  "F2_PCC"
  F2_CB_4/1 -> [F2_CB_4]
  [RELAY_IN] -> Bus Selector1/1
  Bus Selector1/1 -> F2_CB_4/1  "<F2_CB_4>"
  [RELAY_IN] -> Bus Selector26/1
  Bus Selector26/1 -> F2_CB_18/1  "<F2_CB_18>"
  [F2_CB_18] -> Bus Creator5/18  "F2_CB_18"
  [F2_CB_19] -> Bus Creator5/19  "F2_CB_19"
  F2_CB_19/1 -> [F2_CB_19]
  [RELAY_IN] -> Bus Selector27/1
  Bus Selector27/1 -> F2_CB_19/1  "<F2_CB_19>"
  SC_CMD/1 -> OpComm2/1
  Memory/1 -> DATA_OUT/1
  OpComm2/1 -> Bus Selector28/1
  Bus Creator2/1 -> Memory/1
  Bus Creator5/1 -> [CB_DATA]
  [CB_DATA] -> Bus Creator2/1  "CB_DATA"
  [LOAD_DATA] -> Bus Creator2/2  "LOAD_DATA"
  F2_CB_18/1 -> [F2_CB_18]
  [RELAY_IN] -> Bus Selector36/1
  Bus Selector36/1 -> F2_PCC/1  "<F2_PCC>"
  [ESS_DATA] -> Bus Creator2/3  "ESS_DATA"
  [PV_DATA] -> Bus Creator2/4  "PV_DATA"
  Bus Selector28/1 -> [ESS]  "<ESS1_ctrl>"
  Bus Selector28/2 -> [PV]  "<PV1_ctrl>"
  PV1_Modbus/1 -> PV2/1(modbus_in)
  [PV] -> PV2/3(console)
  PV2/1(modbus_out) -> PV1_Modbus/1
  PV2/2(meas) -> [PV_DATA]
  [ESS] -> ESS1/2(console)
  ESS1/2(meas) -> [ESS_DATA]
  ESS1/1(modbus_out) -> ESS1_Modbus/1
  ESS1_Modbus/1 -> ESS1/1(modbus_in)
  OpComm1/1 -> Bus Selector30/1
  Bus Selector30/1 -> [LOAD_IN]  "<LoadProfile>"
  Bus Selector30/2 -> [TestSeq]  "<TestSeq>"
  [TestSeq] -> PV2/2(testseq)
  [TestSeq] -> ESS1/3(testseq)
  connections:
  SSN Interface Block (3ph)2/LConn1 -- C203/RConn1 -- Losses1/LConn3
  SSN Interface Block (3ph)2/LConn2 -- C203/RConn2 -- Losses1/LConn2
  SSN Interface Block (3ph)2/LConn3 -- C203/RConn3 -- Losses1/LConn1
  F2_CB_13/LConn1 -- 1000 kVA1/RConn1 -- Losses5/LConn1 -- F2_CB_12/LConn1
  F2_CB_13/LConn2 -- 1000 kVA1/RConn2 -- Losses5/LConn2 -- F2_CB_12/LConn2
  Losses5/LConn3 -- F2_CB_13/LConn3 -- 1000 kVA1/RConn3 -- F2_CB_12/LConn3
  F2_CB_12/RConn3 -- Interruptible_5/LConn3
  F2_CB_12/RConn2 -- Interruptible_5/LConn2
  F2_CB_12/RConn1 -- Interruptible_5/LConn1
  1000 kVA1/LConn1 -- SSN Interface Block (3ph)9/RConn1
  1000 kVA1/LConn3 -- SSN Interface Block (3ph)9/RConn3
  1000 kVA1/LConn2 -- SSN Interface Block (3ph)9/RConn2
  F2_CB_8/RConn3 -- 1000 kVA2/LConn3
  F2_CB_8/RConn1 -- 1000 kVA2/LConn1
  F2_CB_8/RConn2 -- 1000 kVA2/LConn2
  SSN Interface Block (3ph)4/RConn3 -- F2_CB_3/LConn3
  SSN Interface Block (3ph)4/RConn1 -- F2_CB_3/LConn1
  SSN Interface Block (3ph)4/RConn2 -- F2_CB_3/LConn2
  F2_CB_14/RConn3 -- 2000 kVA2/LConn3
  F2_CB_16/LConn2 -- Losses2/LConn2 -- 2000 kVA3/RConn2 -- F2_CB_18/LConn2
  F2_CB_14/RConn2 -- 2000 kVA2/LConn2
  F2_CB_6/RConn2 -- 500 kVA/LConn2
  SSN Interface Block (3ph)9/LConn3 -- F2_CB_10/RConn3
  F2_CB_9/RConn3 -- 2500 kVA1/LConn3
  C202/RConn3 -- F2_CB_11/LConn3 -- Losses3/LConn3 -- SSN Interface Block (3ph)3/LConn3 -- F2_CB_10/LConn3
  F2_CB_6/RConn3 -- 500 kVA/LConn3
  F2_CB_16/LConn3 -- Losses2/LConn3 -- 2000 kVA3/RConn3 -- F2_CB_18/LConn3
  F2_CB_11/RConn2 -- 5000 kVA/LConn2 -- Losses4/LConn2
  Critical_4/LConn1 -- F2_CB_17/LConn1 -- 2000 kVA2/RConn1
  C202/RConn2 -- F2_CB_11/LConn2 -- Losses3/LConn2 -- F2_CB_10/LConn2 -- SSN Interface Block (3ph)3/LConn2
  4/0AWG-Mutual/LConn1 -- 500kcmil-Mutual8/RConn1 -- SSN Interface Block (3ph)4/LConn1 -- Losses6/LConn3
  3750 kVA/LConn3 -- F2_CB_7/RConn3
  C203/LConn3 -- F2_CB_3/RConn3
  C203/LConn1 -- F2_CB_3/RConn1
  SSN Interface Block (3ph)9/LConn2 -- F2_CB_10/RConn2
  2500 kVA/LConn1 -- F2_CB_5/RConn1
  2500 kVA/LConn3 -- F2_CB_5/RConn3
  2500 kVA/LConn2 -- F2_CB_5/RConn2
  F2_CB_16/LConn1 -- 2000 kVA3/RConn1 -- Losses2/LConn1 -- F2_CB_18/LConn1
  SSN Interface Block (3ph)9/LConn1 -- F2_CB_10/RConn1
  F2_CB_14/RConn1 -- 2000 kVA2/LConn1
  F2_CB_15/RConn1 -- 2000 kVA3/LConn1
  Critical_4/LConn3 -- 2000 kVA2/RConn3 -- F2_CB_17/LConn3
  F2_CB_11/RConn1 -- 5000 kVA/LConn1 -- Losses4/LConn1
  F2_CB_15/RConn3 -- 2000 kVA3/LConn3
  F2_CB_9/RConn1 -- 2500 kVA1/LConn1
  F2_CB_19/LConn2 -- 2500 kVA1/RConn2
  C203/LConn2 -- F2_CB_3/RConn2
  F2_CB_11/RConn3 -- 5000 kVA/LConn3 -- Losses4/LConn3
  Critical_4/LConn2 -- F2_CB_17/LConn2 -- 2000 kVA2/RConn2
  3750 kVA/LConn2 -- F2_CB_7/RConn2
  3750 kVA/LConn1 -- F2_CB_7/RConn1
  F2_CB_11/LConn1 -- SSN Interface Block (3ph)3/LConn1 -- F2_CB_10/LConn1 -- C202/RConn1 -- Losses3/LConn1
  F2_CB_15/RConn2 -- 2000 kVA3/LConn2
  F2_CB_6/RConn1 -- 500 kVA/LConn1
  SSN Interface Block (3ph)4/LConn2 -- 4/0AWG-Mutual/LConn2 -- 500kcmil-Mutual8/RConn2 -- Losses6/LConn2
  500kcmil-Mutual8/RConn3 -- 4/0AWG-Mutual/LConn3 -- SSN Interface Block (3ph)4/LConn3 -- Losses6/LConn1
  F2_CB_9/RConn2 -- 2500 kVA1/LConn2
  F2_CB_19/LConn1 -- 2500 kVA1/RConn1
  F2_CB_19/LConn3 -- 2500 kVA1/RConn3
  F2_CB_18/RConn2 -- Priority_5/LConn2
  F2_CB_18/RConn3 -- Priority_5/LConn3
  F2_CB_19/RConn1 -- Priority_2/LConn1
  F2_CB_19/RConn2 -- Priority_2/LConn2
  F2_CB_19/RConn3 -- Priority_2/LConn3
  SSN Interface Block (3ph)3/RConn2 -- F2_CB_9/LConn2
  SSN Interface Block (3ph)3/RConn3 -- F2_CB_9/LConn3
  SSN Interface Block (3ph)3/RConn1 -- F2_CB_9/LConn1
  C204/LConn3 -- F2_CB_16/RConn3
  C204/LConn1 -- F2_CB_16/RConn1
  C204/LConn2 -- F2_CB_16/RConn2
  C_CB_16/RConn1 -- C204/RConn3 -- 6 kvar inductor at 480V  to cancel kvar produced by the stublines1/LConn3
  B_CB_16/RConn1 -- C204/RConn2 -- 6 kvar inductor at 480V  to cancel kvar produced by the stublines1/LConn2
  A_CB_16/RConn1 -- C204/RConn1 -- 6 kvar inductor at 480V  to cancel kvar produced by the stublines1/LConn1
  C205/LConn3 -- F2_CB_17/RConn3
  C205/LConn1 -- F2_CB_17/RConn1
  C205/LConn2 -- F2_CB_17/RConn2
  C_CB_17/RConn1 -- C205/RConn3 -- 6 kvar inductor at 480V  to cancel kvar produced by the stublines2/LConn3
  B_CB_17/RConn1 -- C205/RConn2 -- 6 kvar inductor at 480V  to cancel kvar produced by the stublines2/LConn2
  A_CB_17/RConn1 -- C205/RConn1 -- 6 kvar inductor at 480V  to cancel kvar produced by the stublines2/LConn1
  C206/LConn3 -- F2_CB_13/RConn3
  C206/LConn2 -- F2_CB_13/RConn2
  C206/LConn1 -- F2_CB_13/RConn1
  C_CB_13/RConn1 -- C206/RConn3 -- 6 kvar inductor at 480V  to cancel kvar produced by the stublines3/LConn3
  B_CB_13/RConn1 -- C206/RConn2 -- 6 kvar inductor at 480V  to cancel kvar produced by the stublines3/LConn2
  A_CB_13/RConn1 -- C206/RConn1 -- 6 kvar inductor at 480V  to cancel kvar produced by the stublines3/LConn1
  1500 kVA/RConn3 -- Priority_3/LConn3
  1500 kVA/RConn2 -- Priority_3/LConn2
  1500 kVA/RConn1 -- Priority_3/LConn1
  F2_CB_4/RConn3 -- 1500 kVA/LConn3
  F2_CB_4/RConn2 -- 1500 kVA/LConn2
  F2_CB_4/RConn1 -- 1500 kVA/LConn1
  SSN Interface Block (3ph)4/RConn5 -- F2_CB_2/LConn2
  SSN Interface Block (3ph)4/RConn6 -- F2_CB_2/LConn3
  SSN Interface Block (3ph)4/RConn4 -- F2_CB_2/LConn1
  C202/LConn2 -- F2_CB_2/RConn2
  C202/LConn1 -- F2_CB_2/RConn1
  C202/LConn3 -- F2_CB_2/RConn3
  SSN Interface Block (3ph)2/RConn1 -- F2_CB_15/LConn1
  SSN Interface Block (3ph)2/RConn2 -- F2_CB_15/LConn2
  SSN Interface Block (3ph)2/RConn3 -- F2_CB_15/LConn3
  SSN Interface Block (3ph)2/RConn6 -- F2_CB_14/LConn3
  SSN Interface Block (3ph)2/RConn5 -- F2_CB_14/LConn2
  SSN Interface Block (3ph)2/RConn4 -- F2_CB_14/LConn1
  2500 kVA/RConn1 -- ESS1/RConn1 -- Critical_3/LConn1
  2500 kVA/RConn3 -- ESS1/RConn3 -- Critical_3/LConn3
  2500 kVA/RConn2 -- ESS1/RConn2 -- Critical_3/LConn2
  1000 kVA2/RConn1 -- Interruptible_4/LConn1
  1000 kVA2/RConn2 -- Interruptible_4/LConn2
  1000 kVA2/RConn3 -- Interruptible_4/LConn3
  500 kVA/RConn2 -- Interruptible_3/LConn2
  500 kVA/RConn3 -- Interruptible_3/LConn3
  500 kVA/RConn1 -- Interruptible_3/LConn1
  F2_PCC/RConn1 -- 500kcmil-Mutual8/LConn1
  F2_PCC/RConn2 -- 500kcmil-Mutual8/LConn2
  F2_PCC/RConn3 -- 500kcmil-Mutual8/LConn3
  F2_PCC/LConn3 -- 500kcmil-Mutual5/RConn3
  F2_PCC/LConn2 -- 500kcmil-Mutual5/RConn2
  F2_PCC/LConn1 -- 500kcmil-Mutual5/RConn1
  F2_CB_18/RConn1 -- Priority_5/LConn1
  PCC_B/RConn1 -- 448 kvar inductor at 13.8kV  to cancel kvar produced by the stublines1/LConn2 -- 500kcmil-Mutual5/LConn2
  PCC_A/RConn1 -- 448 kvar inductor at 13.8kV  to cancel kvar produced by the stublines1/LConn1 -- 500kcmil-Mutual5/LConn1
  PCC_C/RConn1 -- 448 kvar inductor at 13.8kV  to cancel kvar produced by the stublines1/LConn3 -- 500kcmil-Mutual5/LConn3
  4/0AWG-Mutual/RConn2 -- F2_CB_1/LConn2
  4/0AWG-Mutual/RConn1 -- F2_CB_1/LConn1
  4/0AWG-Mutual/RConn3 -- F2_CB_1/LConn3
  SSN Interface Block (3ph)10/LConn3 -- F2_CB_1/RConn3
  SSN Interface Block (3ph)10/LConn2 -- F2_CB_1/RConn2
  SSN Interface Block (3ph)10/LConn1 -- F2_CB_1/RConn1
  C201/LConn2 -- SSN Interface Block (3ph)10/RConn2
  C201/LConn1 -- SSN Interface Block (3ph)10/RConn1
  C201/LConn3 -- SSN Interface Block (3ph)10/RConn3
  SSN Interface Block (3ph)5/RConn2 -- F2_CB_5/LConn2 -- F2_CB_7/LConn2
  SSN Interface Block (3ph)5/RConn1 -- F2_CB_5/LConn1 -- F2_CB_7/LConn1
  SSN Interface Block (3ph)5/RConn3 -- F2_CB_5/LConn3 -- F2_CB_7/LConn3
  SSN Interface Block (3ph)1/LConn3 -- 3750 kVA/RConn3
  SSN Interface Block (3ph)1/LConn2 -- 3750 kVA/RConn2
  SSN Interface Block (3ph)1/LConn1 -- 3750 kVA/RConn1
  PV2/RConn1 -- 5000 kVA/RConn1
  PV2/RConn3 -- 5000 kVA/RConn3
  PV2/RConn2 -- 5000 kVA/RConn2
  SSN Interface Block (3ph)5/LConn3 -- F2_CB_6/LConn3 -- C201/RConn3 -- Losses8/LConn1
  SSN Interface Block (3ph)5/LConn1 -- F2_CB_6/LConn1 -- C201/RConn1 -- Losses8/LConn3
  SSN Interface Block (3ph)5/LConn2 -- F2_CB_6/LConn2 -- C201/RConn2 -- Losses8/LConn2
  F2_CB_4/LConn3 -- SSN Interface Block (3ph)1/RConn3 -- Losses7/LConn3 -- F2_CB_8/LConn3
  F2_CB_4/LConn2 -- SSN Interface Block (3ph)1/RConn2 -- Losses7/LConn2 -- F2_CB_8/LConn2
  F2_CB_4/LConn1 -- SSN Interface Block (3ph)1/RConn1 -- Losses7/LConn1 -- F2_CB_8/LConn1
